simulink model "base_active_suspension"  (R2020a)
settings: Solver=ode23tb  StartTime=0.0  StopTime=simlength  MaxStep=Tc
values from neighbouring files (symbols this model uses):
  L = L'    [init_active_suspension.m]
  Tc = 1e-5    (= 1e-05)    [init_active_suspension.m]
  time_spd_b_on = 1    [init_active_suspension.m]
libraries: nesl_utility x7, fl_lib x4, cstblocks x1, suspension_single_mass_lib x1
settings Model: SimulationMode=accelerator  Creator=dbagn  LastModifiedBy=dbagn
settings DataIOCC: ReturnWorkspaceOutputs=off

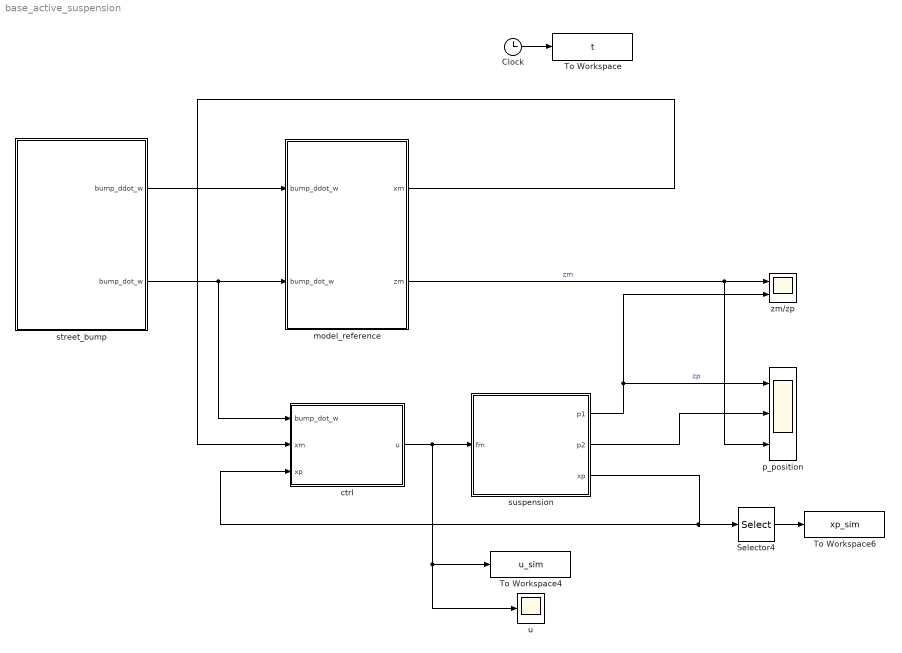
== system base_active_suspension ==
  Clock : Clock
  Selector4 : Selector  InputPortWidth=2  IndexOptions=Index vector (dialog)  Indices=1  OutputSizes=1
  To Workspace : ToWorkspace  VariableName=t  SampleTime=Tc
      settings: MaxDataPoints=Nc
  To Workspace4 : ToWorkspace  VariableName=u_sim  SampleTime=Tc
      settings: MaxDataPoints=Nc
  To Workspace6 : ToWorkspace  VariableName=xp_sim  SampleTime=Tc
      settings: MaxDataPoints=Nc
  ctrl : Subsystem
  model_reference : Subsystem
  p_position : Scope  NumInputPorts=3
  street_bump : Subsystem
  suspension : Subsystem
  u : Scope
  zm/zp : Scope  NumInputPorts=2
  wires:
  suspension/1(p1) -> p_position/1, zm/zp/2  "zp"
  model_reference/1(xm) -> ctrl/2(xm)
  ctrl/1(u) -> u/1, To Workspace4/1, suspension/1(fm)
  suspension/3(xp) -> Selector4/1, ctrl/3(xp)
  model_reference/2(zm) -> zm/zp/1, p_position/3  "zm"
  suspension/2(p2) -> p_position/2
  Clock/1 -> To Workspace/1
  Selector4/1 -> To Workspace6/1
  street_bump/1(bump_ddot_w) -> model_reference/1(bump_ddot_w)
  street_bump/2(bump_dot_w) -> ctrl/1(bump_dot_w), model_reference/2(bump_dot_w)

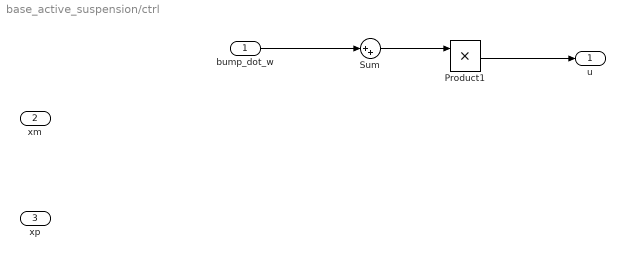
== system base_active_suspension/ctrl ==
  bump_dot_w : Inport
  xm : Inport  Port=2
  xp : Inport  Port=3
  Product1 : Product
  Sum : Sum  Inputs=|++
  u : Outport
  wires:
  Sum/1 -> Product1/1
  Product1/1 -> u/1
  bump_dot_w/1 -> Sum/1

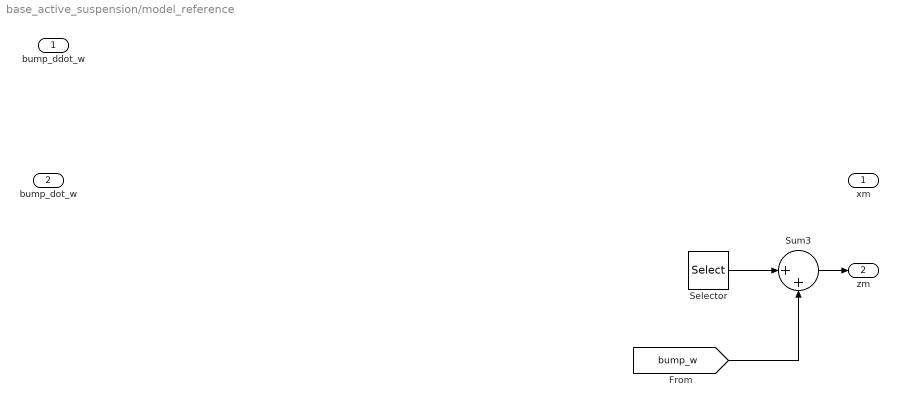
== system base_active_suspension/model_reference ==
  bump_ddot_w : Inport
  bump_dot_w : Inport  Port=2
  Selector : Selector  InputPortWidth=2  IndexOptions=Index vector (dialog)  Indices=1  OutputSizes=1
  Sum3 : Sum  Inputs=|++
  xm : Outport
  zm : Outport  Port=2
  wires:
  ? -> Selector/1, xm/1
  Sum3/1 -> zm/1
  [bump_w] -> Sum3/2
  Selector/1 -> Sum3/1

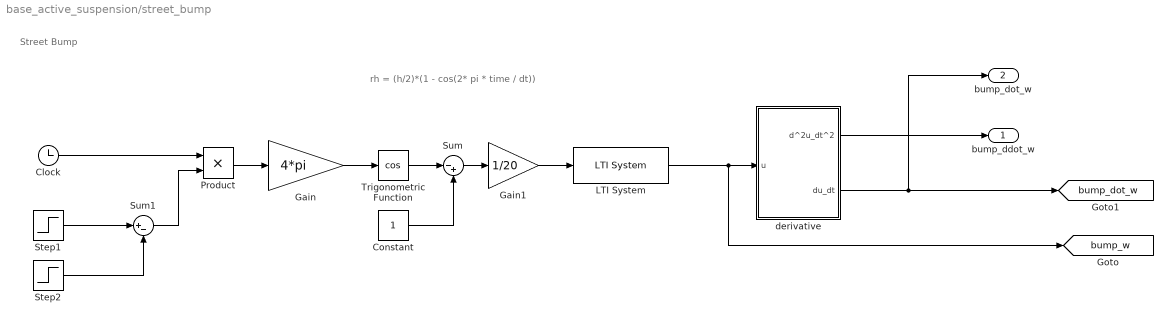
== system base_active_suspension/street_bump ==
  note: Street Bump
  note: rh = (h/2)*(1 - cos(2* pi * time / dt))
  Clock : Clock
  Constant : Constant
  Gain : Gain  Gain=4*pi
  Gain1 : Gain  Gain=1/20
  LTI System : cstblocks/LTI System  sys=spd_bump_flt_ss  IC=spd_bump_flt_init
  Product : Product
  Step1 : Step  Time=time_spd_b_on  SampleTime=0
  Step2 : Step  Time=time_spd_b_on+0.5  SampleTime=0
  Sum : Sum  Inputs=|-+
  Sum1 : Sum  Inputs=|+-
  Trigonometric Function : Trigonometry  Operator=cos
  derivative : Subsystem
  bump_ddot_w : Outport
  bump_dot_w : Outport  Port=2
  tag scope: bump_dot_w=global, bump_w=global
  wires:
  Gain/1 -> Trigonometric Function/1
  Trigonometric Function/1 -> Sum/1
  Constant/1 -> Sum/2
  Sum/1 -> Gain1/1
  Clock/1 -> Product/1
  Product/1 -> Gain/1
  Step1/1 -> Sum1/1
  Sum1/1 -> Product/2
  Step2/1 -> Sum1/2
  Gain1/1 -> LTI System/1
  LTI System/1 -> derivative/1(u), [bump_w]
  derivative/1(d^2u_dt^2) -> bump_ddot_w/1
  derivative/2(du_dt) -> bump_dot_w/1, [bump_dot_w]

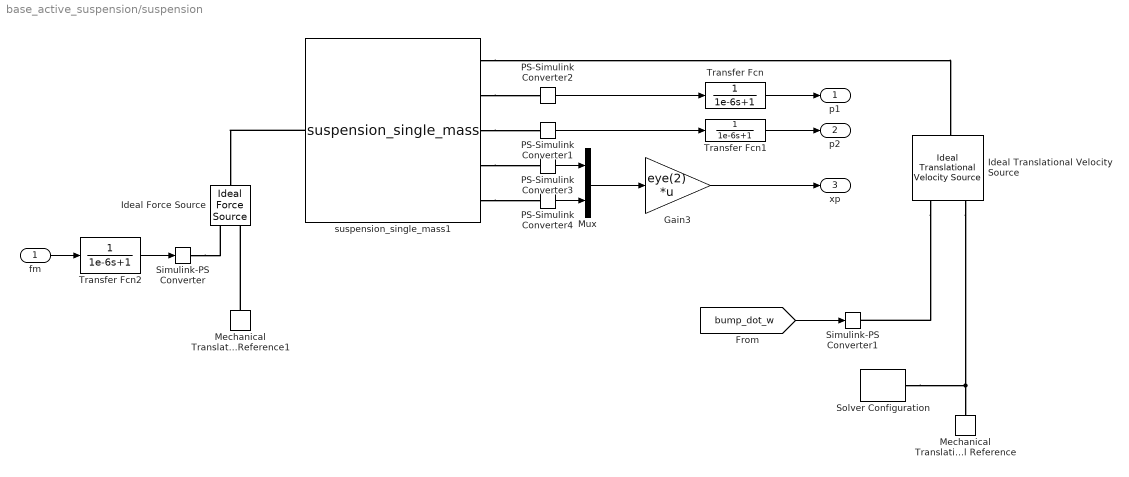
== system base_active_suspension/suspension ==
  fm : Inport
  Gain3 : Gain  Gain=eye(2)  Multiplication=Matrix(K*u)
  Ideal Force Source : fl_lib/Mechanical/Mechanical Sources/Ideal Force Source
  Ideal Translational Velocity Source : fl_lib/Mechanical/Mechanical Sources/Ideal Translational Velocity Source
  Mechanical Translational Reference : fl_lib/Mechanical/Translational Elements/Mechanical Translational Reference
  Mechanical Translational Reference1 : fl_lib/Mechanical/Translational Elements/Mechanical Translational Reference
  Mux : Mux  Inputs=2
  PS-Simulink Converter{1..4} (4 alike) : nesl_utility/PS-Simulink Converter  PhysicalDomain=network_engine_domain  SubClassName=ps_output  LeftPortType=input  RightPortType=output  PseudoPeriodic=off  Frequencies=[]  Unit=inherit  AffineConversion=off
  Simulink-PS Converter : nesl_utility/Simulink-PS Converter  PhysicalDomain=network_engine_domain  SubClassName=ps_input  LeftPortType=input  RightPortType=output  PseudoPeriodic=off  Frequencies=[]  NoiseDistribution=none  NoiseParameters=[]  Unit=1  AffineConversion=off  FilteringAndDerivatives=provide  SimscapeFilterOrder=1  InputFilterTimeConstant=0.001  UdotUserProvided=0
  Simulink-PS Converter1 : nesl_utility/Simulink-PS Converter  PhysicalDomain=network_engine_domain  SubClassName=ps_input  LeftPortType=input  RightPortType=output  PseudoPeriodic=off  Frequencies=[]  NoiseDistribution=none  NoiseParameters=[]  Unit=1  AffineConversion=off  FilteringAndDerivatives=provide  SimscapeFilterOrder=1  InputFilterTimeConstant=0.001  UdotUserProvided=0
  Solver Configuration : nesl_utility/Solver Configuration  PhysicalDomain=network_engine_domain  SubClassName=solver  LeftPortType=input  RightPortType=generic  Tones=[]  Harmonics=[]  SimulateNoise=off  Profile=off  UseLocalSampling=off  EnableSwitchedLinearOptims=on  FrequencyDomain=off  UseCCode=off  RelTol=0.001  AbsTol=1e-06  MinStep=1e-09  ToWorkspace=off  RevertToSquareIcSolve=off  NumHomotopyIterations=100  PhasorMode=off  PhasorModeNumHarmonics=1  DoDC=off  ResidualTolerance=1e-09  UseLocalSolver=on  LocalSolverChoice=NE_BACKWARD_EULER_ADVANCER  LocalSolverSampleTime=Ts  DoFixedCost=on  MaxNonlinIter=3  MaxModeIter=2  LinearAlgebra=auto  EquationFormulation=NE_TIME_EF  DelaysMemoryBudget=1024  AutomaticFiltering=on  FilteringTimeConstant=0.001  PartitionStorageMethod=AS_NEEDED  PartitionMemoryBudget=1024  PartitionMethod=ROBUST
  Transfer Fcn : TransferFcn  Denominator=[1e-6 1]
  Transfer Fcn1 : TransferFcn  Denominator=[1e-6 1]
  Transfer Fcn2 : TransferFcn  Denominator=[1e-6 1]
  suspension_single_mass1 : suspension_single_mass_lib/suspension_single_mass  mp=mp kg  kp=kp N/m  bp=bp N/(m/s)  x0=x0 m
      settings: InternalSimscapePortConfiguration="{\"Bottom\":[],\"Left\":[{\"id\":\"P1\",\"label\":\"P1\",\"type\":\"foundation.mechanical.translational.translational\"}],\"Right\":[{\"id\":\"P2\",\"label\":\"P2\",\"type\":\"foundation.mechanical.translational.translational\"},{\"id\":\"p1\",\"label\":\"p1\",\"type\":\"output\"},{\"id\":\"p2\",\"label\":\"p2\",\"type\":\"output\"},{\"id\":\"x\",\"label\":\"x\",\"type\":\"output\"},{\"id\":\"x_dot\",\"label\":\"x_dot\",\"type\":\"output\"}],\"Top\":[]}"
  p1 : Outport
  p2 : Outport  Port=2
  xp : Outport  Port=3
  wires:
  PS-Simulink Converter1/1 -> Transfer Fcn1/1
  fm/1 -> Transfer Fcn2/1
  [bump_dot_w] -> Simulink-PS Converter1/1
  PS-Simulink Converter2/1 -> Transfer Fcn/1
  PS-Simulink Converter3/1 -> Mux/1
  PS-Simulink Converter4/1 -> Mux/2
  Transfer Fcn/1 -> p1/1
  Transfer Fcn1/1 -> p2/1
  Mux/1 -> Gain3/1
  Transfer Fcn2/1 -> Simulink-PS Converter/1
  Gain3/1 -> xp/1
  connections:
  suspension_single_mass1/RConn1 -- Ideal Translational Velocity Source/LConn1
  Mechanical Translational Reference1/LConn1 -- Ideal Force Source/RConn2
  suspension_single_mass1/LConn1 -- Ideal Force Source/LConn1
  Simulink-PS Converter/RConn1 -- Ideal Force Source/RConn1
  Ideal Translational Velocity Source/RConn1 -- Simulink-PS Converter1/RConn1
  Solver Configuration/RConn1 -- Mechanical Translational Reference/LConn1 -- Ideal Translational Velocity Source/RConn2
  suspension_single_mass1/RConn3 -- PS-Simulink Converter1/LConn1
  suspension_single_mass1/RConn2 -- PS-Simulink Converter2/LConn1
  suspension_single_mass1/RConn4 -- PS-Simulink Converter3/LConn1
  suspension_single_mass1/RConn5 -- PS-Simulink Converter4/LConn1

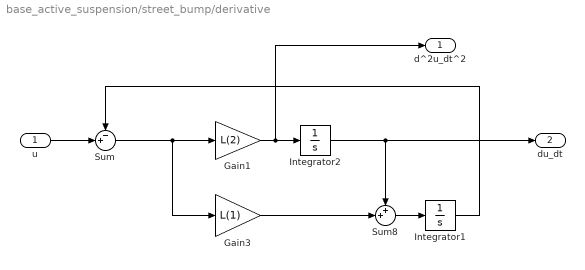
== system base_active_suspension/street_bump/derivative ==
  u : Inport
  Gain1 : Gain  Gain=L(2)
  Gain3 : Gain  Gain=L(1)
  Integrator1 : Integrator
  Integrator2 : Integrator
  Sum : Sum  Inputs=-+|
  Sum8 : Sum  Inputs=++|
  d^2u_dt^2 : Outport  VectorParamsAs1DForOutWhenUnconnected=off
  du_dt : Outport  Port=2  VectorParamsAs1DForOutWhenUnconnected=off
  wires:
  Sum8/1 -> Integrator1/1
  u/1 -> Sum/2
  Integrator1/1 -> Sum/1
  Gain1/1 -> d^2u_dt^2/1, Integrator2/1
  Sum/1 -> Gain3/1, Gain1/1
  Gain3/1 -> Sum8/2
  Integrator2/1 -> du_dt/1, Sum8/1
